simulink model "LaserLiFiSimulation"  (R2025b)
settings: Solver=VariableStepAuto  StartTime=0.0  StopTime=10  RelTol=1e-3

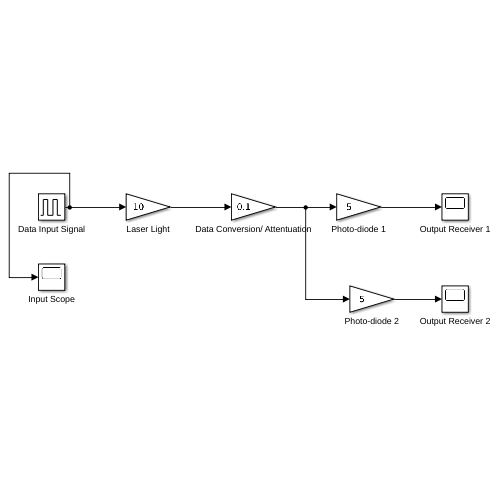
[thumbnail: Simulink's stored preview of the top-level diagram]
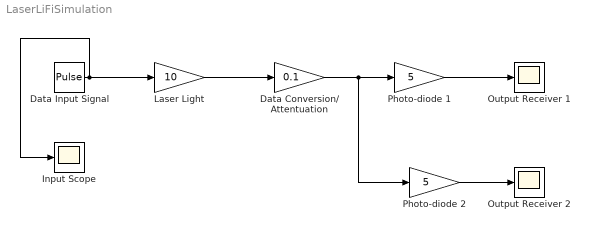
== system LaserLiFiSimulation ==
  Data Conversion/ Attentuation : Gain  Gain=0.1
  Data Input Signal : DiscretePulseGenerator  PulseType=Time based  Period=1  PulseWidth=50
  Input Scope : Scope
      settings: ActiveDisplayYMinimum=-0.12499999999999997  ActiveDisplayYMaximum=1.125
  Laser Light : Gain  Gain=10
  Output Receiver 1 : Scope
      settings: ActiveDisplayYMinimum=-0.62499999999999989  ActiveDisplayYMaximum=5.625
  Output Receiver 2 : Scope
      settings: ActiveDisplayYMinimum=-0.62499999999999989  ActiveDisplayYMaximum=5.625
  Photo-diode 1 : Gain  Gain=5
  Photo-diode 2 : Gain  Gain=5
  wires:
  Data Input Signal/1 -> Laser Light/1, Input Scope/1
  Laser Light/1 -> Data Conversion/ Attentuation/1
  Data Conversion/ Attentuation/1 -> Photo-diode 1/1, Photo-diode 2/1
  Photo-diode 1/1 -> Output Receiver 1/1
  Photo-diode 2/1 -> Output Receiver 2/1
